simulink model "GSM_Netzwerk"  (R2017b)
settings: Solver=VariableStepAuto  StartTime=0.0  StopTime=10  RelTol=1e-3
values from neighbouring files (symbols this model uses):
  A = double(A)    [GSM_Parameter.m]
  A_red = double(A_red)    [GSM_Parameter.m]
  Ad = RzSS.a    [GSM_Parameter.m]
  AdPI = RzPISS.a    [GSM_Parameter.m]
  B = [double(Bu) double(Bd)]    [GSM_Parameter.m]
  B_red = [double(Bu_red) double(Bd_red)]    [GSM_Parameter.m]
  Bd = RzSS.b    [GSM_Parameter.m]
  BdPI = RzPISS.b    [GSM_Parameter.m]
  Cd = RzSS.c    [GSM_Parameter.m]
  CdPI = RzPISS.c    [GSM_Parameter.m]
  cGSMP = 0.6822    [GSM_Parameter.m]
  dcGSM = 0.152    [GSM_Parameter.m]
  dcP = 0.169    [GSM_Parameter.m]
  Dd = RzSS.d    [GSM_Parameter.m]
  DdPI = RzPISS.d    [GSM_Parameter.m]
  dGSMP = 1e-5    (= 1e-05)    [GSM_Parameter.m]
  dqP = 1e-4    (= 0.0001)    [GSM_Parameter.m]
  dvGSM = 1.8e-3    (= 0.0018)    [GSM_Parameter.m]
  dvP = 2.7e-3    (= 0.0027)    [GSM_Parameter.m]
  iGSM_0 = ruhelage(2,1)    [GSM_Parameter.m]
  JGSM = 12.4e-3    (= 0.0124)    [GSM_Parameter.m]
  JP = 32.5e-3    (= 0.0325)    [GSM_Parameter.m]
  kGSM = 0.1    [GSM_Parameter.m]
  LGSM = 1.4e-3    (= 0.0014)    [GSM_Parameter.m]
  MextR = 0    [GSM_Parameter.m]
  phiGSMP_0 = ruhelage(2,2)    [GSM_Parameter.m]
  RGSM = 0.46    [GSM_Parameter.m]
  Ta = 10e-3    (= 0.01)    [GSM_Parameter.m]
  uGSMR = 5.6    [GSM_Parameter.m]
  wGSM_0 = ruhelage(2,3)    [GSM_Parameter.m]
  wP_0 = ruhelage(2,4)    [GSM_Parameter.m]
settings Model: Creator=user  LastModifiedBy=user
settings SFSimCC: SimUseLocalCustomCode=on
settings RTWCC: RTWUseLocalCustomCode=on

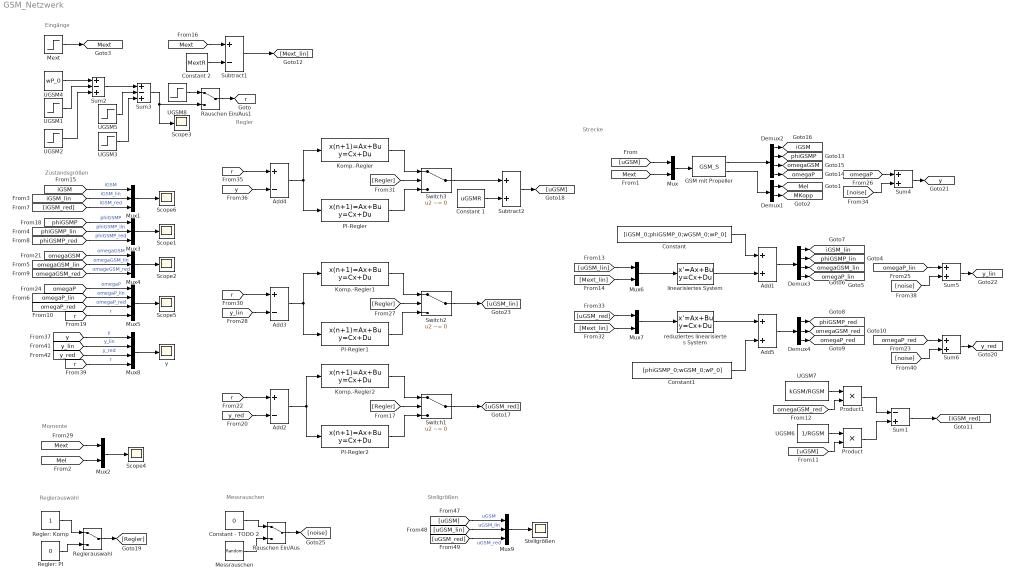
== system GSM_Netzwerk ==
  note: Eingänge
  note: Momente
  note: Reglerauswahl
  note: Zustandsgrößen
  note: Strecke
  note: Messrauschen
  note: Stellgrößen
  note: Regler
  Add1 : Sum
  Add2 : Sum  Inputs=+-
  Add3 : Sum  Inputs=+-
  Add4 : Sum  Inputs=+-
  Add5 : Sum
  Constant : Constant  Value=[iGSM_0;phiGSMP_0;wGSM_0;wP_0]
  Constant - TODO 2 : Constant  Value=0
  Constant 1 : Constant  Value=uGSMR
  Constant 2 : Constant  Value=MextR
  Constant1 : Constant  Value=[phiGSMP_0;wGSM_0;wP_0]
  Demux1 : Demux  Outputs=2
  Demux2 : Demux
  Demux3 : Demux
  Demux4 : Demux  Outputs=3
  GSM mit Propeller : M-S-Function  FunctionName=GSM_S  Parameters=iGSM_0, qGSMP_0, wGSM_0, wP_0, LGSM, RGSM, kGSM, JGSM, dcGSM, dvGSM, JP, dcP, dvP, dqP, cGSMP, dGSMP  mask{iGSM_0=iGSM_0, qGSMP_0=phiGSMP_0, wGSM_0=wGSM_0, wP_0=wP_0, LGSM=LGSM, RGSM=RGSM, kGSM=kGSM, JGSM=JGSM, dcGSM=dcGSM, dvGSM=dvGSM, JP=JP, dcP=dcP, dvP=dvP, dqP=dqP, cGSMP=cGSMP, dGSMP=dGSMP}
  Komp.-Regler : DiscreteStateSpace  A=Ad  B=Bd  C=Cd  D=Dd  SampleTime=Ta
  Komp.-Regler1 : DiscreteStateSpace  A=Ad  B=Bd  C=Cd  D=Dd  SampleTime=Ta
  Komp.-Regler2 : DiscreteStateSpace  A=Ad  B=Bd  C=Cd  D=Dd  SampleTime=Ta
  Messrauschen : UniformRandomNumber  Minimum=-5e-2  Maximum=5e-2  SampleTime=1e-3
  Mext : Step  Time=11  After=0.25  SampleTime=0
  Mux{,2,6..7} (4 alike) : Mux  Inputs=2
  Mux{1,3..4,9} (4 alike) : Mux  Inputs=3
  Mux5 : Mux
  Mux8 : Mux
  PI-Regler : DiscreteStateSpace  A=AdPI  B=BdPI  C=CdPI  D=DdPI  SampleTime=Ta
  PI-Regler1 : DiscreteStateSpace  A=AdPI  B=BdPI  C=CdPI  D=DdPI  SampleTime=Ta
  PI-Regler2 : DiscreteStateSpace  A=AdPI  B=BdPI  C=CdPI  D=DdPI  SampleTime=Ta
  Product : Product
  Product1 : Product
  Rauschen Ein/Aus : ManualSwitch
  Rauschen Ein/Aus1 : ManualSwitch
  Regler: Komp : Constant
  Regler: PI : Constant  Value=0
  Reglerauswahl : ManualSwitch
  Scope{1..6} (6 alike) : Scope
  Stellgrößen : Scope
  Subtract1 : Sum  Inputs=+-
  Subtract2 : Sum
  Sum1 : Sum  Inputs=-+
  Sum2 : Sum  Inputs=+-+
  Sum3 : Sum  Inputs=+-+
  Sum4 : Sum
  Sum5 : Sum
  Sum6 : Sum
  Switch1 : Switch  Criteria=u2 ~= 0
  Switch2 : Switch  Criteria=u2 ~= 0
  Switch3 : Switch  Criteria=u2 ~= 0
  UGSM1 : Step  Time=2  SampleTime=0
  UGSM2 : Step  Time=5  SampleTime=0
  UGSM3 : Step  Time=13  After=2  SampleTime=0
  UGSM4 : Constant  Value=wP_0
  UGSM5 : Step  Time=8  After=2  SampleTime=0
  UGSM6 : Constant  Value=1/RGSM
  UGSM7 : Constant  Value=kGSM/RGSM
  UGSM8 : Step  Time=2  After=wP_0+20  SampleTime=0
  "linearisiertes System " : StateSpace  A=A  B=B  C=eye(4)  D=zeros(4,2)  InitialCondition=[0, 0, 0, 0]
  reduziertes linearisiertes System : StateSpace  A=A_red  B=B_red  C=eye(3)  D=zeros(3,2)  InitialCondition=[0, 0, 0]
  y : Scope
  tag scope: MKopp=global, Mel=global, Mext=global, iGSM=global, iGSM_lin=global, omegaGSM=global, omegaGSM_lin=global, omegaGSM_red=global, omegaP=global, omegaP_lin=global, omegaP_red=global, phiGSMP=global, phiGSMP_lin=global, phiGSMP_red=global, r=global, y=global, y_lin=global, y_red=global
  wires:
  [Mext_lin] -> Mux7/2
  Constant/1 -> Add1/1
  [y_lin] -> Mux8/2  "y_lin"
  Messrauschen/1 -> Rauschen Ein/Aus/2
  Komp.-Regler1/1 -> Switch2/1
  PI-Regler2/1 -> Switch1/3
  [uGSM_lin] -> Mux9/2  "uGSM_lin"
  UGSM2/1 -> Sum2/3
  [r] -> Mux8/4  "r"
  [uGSM_lin] -> Mux6/1
  PI-Regler1/1 -> Switch2/3
  Mux4/1 -> Scope2/1
  Regler: Komp/1 -> Reglerauswahl/1
  UGSM5/1 -> Sum3/2
  Reglerauswahl/1 -> [Regler]
  Komp.-Regler2/1 -> Switch1/1
  [phiGSMP_lin] -> Mux3/2  "phiGSMP_lin"
  reduziertes linearisiertes System/1 -> Add5/1
  Rauschen Ein/Aus/1 -> [noise]
  Sum4/1 -> [y]
  [y_red] -> Mux8/3  "y_red"
  Product1/1 -> Sum1/1
  Constant - TODO 2/1 -> Rauschen Ein/Aus/1
  [noise] -> Sum5/2
  Demux1/2 -> [MKopp]
  [omegaP_lin] -> Sum5/1
  [y_red] -> Add2/2
  Sum5/1 -> [y_lin]
  [omegaP_red] -> Sum6/1
  Sum2/1 -> Sum3/1
  [omegaP] -> Sum4/1
  [r] -> Add4/1
  [r] -> Mux5/4  "r"
  Demux4/1 -> [phiGSMP_red]
  [noise] -> Sum4/2
  [Regler] -> Switch3/2
  [omegaP] -> Mux5/1  "omegaP"
  Add5/1 -> Demux4/1
  [Mext] -> Subtract1/1
  Demux3/3 -> [omegaGSM_lin]
  Demux4/3 -> [omegaP_red]
  [Regler] -> Switch2/2
  Subtract2/1 -> [uGSM]
  PI-Regler/1 -> Switch3/3
  Add4/1 -> PI-Regler/1, Komp.-Regler/1
  [r] -> Add3/1
  Add3/1 -> PI-Regler1/1, Komp.-Regler1/1
  [Mel] -> Mux2/2
  [Regler] -> Switch1/2
  [uGSM_red] -> Mux7/1
  [omegaGSM] -> Mux4/1  "omegaGSM"
  Mux6/1 -> "linearisiertes System "/1
  [r] -> Add2/1
  Demux3/2 -> [phiGSMP_lin]
  [y] -> Add4/2
  Mux5/1 -> Scope5/1
  Switch3/1 -> Subtract2/1
  [iGSM_lin] -> Mux1/2  "iGSM_lin"
  [noise] -> Sum6/2
  UGSM7/1 -> Product1/1
  Switch1/1 -> [uGSM_red]
  [omegaGSM_red] -> Product1/2
  Demux2/3 -> [omegaGSM]
  [Mext] -> Mux/2
  [iGSM] -> Mux1/1  "iGSM"
  [iGSM_red] -> Mux1/3  "iGSM_red"
  GSM mit Propeller/1 -> Demux2/1
  [omegaGSM_red] -> Mux4/3  "omageGSM_red"
  Komp.-Regler/1 -> Switch3/1
  Sum6/1 -> [y_red]
  Add1/1 -> Demux3/1
  [uGSM] -> Mux9/1  "uGSM"
  Demux2/1 -> [iGSM]
  Add2/1 -> PI-Regler2/1, Komp.-Regler2/1
  [uGSM] -> Product/2
  Product/1 -> Sum1/2
  [omegaGSM_lin] -> Mux4/2  "omegaGSM_lin"
  Constant 2/1 -> Subtract1/2
  UGSM1/1 -> Sum2/2
  Mux1/1 -> Scope6/1
  [Mext_lin] -> Mux6/2
  Demux3/4 -> [omegaP_lin]
  Constant1/1 -> Add5/2
  Subtract1/1 -> [Mext_lin]
  UGSM3/1 -> Sum3/3
  Mux8/1 -> y/1
  Demux1/1 -> [Mel]
  Mux/1 -> GSM mit Propeller/1
  Demux2/4 -> [omegaP]
  [phiGSMP] -> Mux3/1  "phiGSMP"
  Sum3/1 -> Scope3/1, Rauschen Ein/Aus1/2
  Mux3/1 -> Scope1/1
  [y] -> Mux8/1  "y"
  [uGSM] -> Mux/1
  Switch2/1 -> [uGSM_lin]
  [Mext] -> Mux2/1
  Constant 1/1 -> Subtract2/2
  Mux7/1 -> reduziertes linearisiertes System/1
  Mux2/1 -> Scope4/1
  Mext/1 -> [Mext]
  UGSM6/1 -> Product/1
  Demux4/2 -> [omegaGSM_red]
  [phiGSMP_red] -> Mux3/3  "phiGSMP_red"
  [omegaP_lin] -> Mux5/2  "omegaP_lin"
  UGSM4/1 -> Sum2/1
  "linearisiertes System "/1 -> Add1/2
  [omegaP_red] -> Mux5/3  "omegaP_red"
  Demux3/1 -> [iGSM_lin]
  Regler: PI/1 -> Reglerauswahl/2
  Sum1/1 -> [iGSM_red]
  [uGSM_red] -> Mux9/3  "uGSM_red"
  [y_lin] -> Add3/2
  Demux2/2 -> [phiGSMP]
  Mux9/1 -> Stellgrößen/1
  GSM mit Propeller/2 -> Demux1/1
  UGSM8/1 -> Rauschen Ein/Aus1/1
  Rauschen Ein/Aus1/1 -> [r]
